simulink model "enginePistonPropC172p"  (R2026a)
settings: Solver=FixedStepAuto  FixedStep=0.004
settings Model: Creator=Edison Altamirano  LastModifiedBy=Edison Altamirano

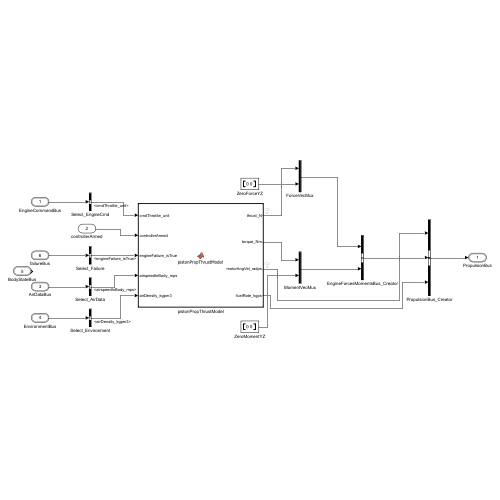
[thumbnail: Simulink's stored preview of the top-level diagram]
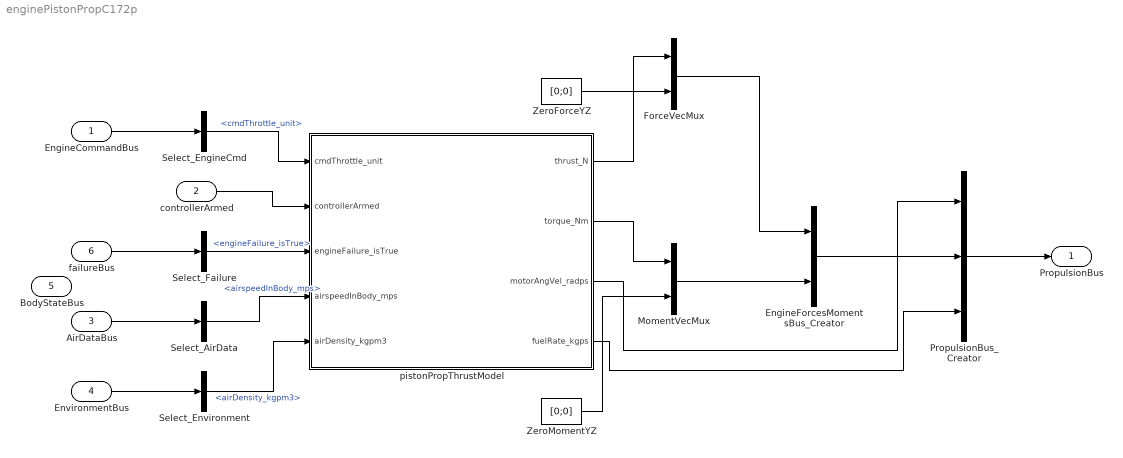
== system enginePistonPropC172p ==
  EngineCommandBus : Inport  OutDataTypeStr=Bus: EngineCommandBus
  controllerArmed : Inport  Port=2
  AirDataBus : Inport  Port=3  OutDataTypeStr=Bus: AirDataBus
  EnvironmentBus : Inport  Port=4  OutDataTypeStr=Bus: EnvironmentBus
  BodyStateBus : Inport  Port=5  OutDataTypeStr=Bus: BodyStateBus
  failureBus : Inport  Port=6  OutDataTypeStr=Bus: FailureBus
  EngineForcesMomentsBus_Creator : BusCreator  Inputs=2  OutDataTypeStr=Bus: ComponentForcesMomentsBus
  ForceVecMux : Mux  Inputs=2
  MomentVecMux : Mux  Inputs=2
  PropulsionBus_Creator : BusCreator  Inputs=3  OutDataTypeStr=Bus: PropulsionBus
  Select_AirData : BusSelector  OutputSignals=airspeedInBody_mps
  Select_EngineCmd : BusSelector  OutputSignals=cmdThrottle_unit
  Select_Environment : BusSelector  OutputSignals=AirEnvironment.airDensity_kgpm3
  Select_Failure : BusSelector  OutputSignals=engineFailure_isTrue
  ZeroForceYZ : Constant  Value=[0;0]
  ZeroMomentYZ : Constant  Value=[0;0]
  pistonPropThrustModel : MATLAB Function  TreatAsAtomicUnit=on
  PropulsionBus : Outport  OutDataTypeStr=Bus: PropulsionBus
  wires:
  EngineCommandBus/1 -> Select_EngineCmd/1
  Select_Failure/1 -> pistonPropThrustModel/3(engineFailure_isTrue)  "<engineFailure_isTrue>"
  AirDataBus/1 -> Select_AirData/1
  EnvironmentBus/1 -> Select_Environment/1
  pistonPropThrustModel/2(torque_Nm) -> MomentVecMux/1
  failureBus/1 -> Select_Failure/1
  Select_EngineCmd/1 -> pistonPropThrustModel/1(cmdThrottle_unit)  "<cmdThrottle_unit>"
  Select_AirData/1 -> pistonPropThrustModel/4(airspeedInBody_mps)  "<airspeedInBody_mps>"
  controllerArmed/1 -> pistonPropThrustModel/2(controllerArmed)
  PropulsionBus_Creator/1 -> PropulsionBus/1
  Select_Environment/1 -> pistonPropThrustModel/5(airDensity_kgpm3)  "<airDensity_kgpm3>"
  ZeroForceYZ/1 -> ForceVecMux/2
  pistonPropThrustModel/1(thrust_N) -> ForceVecMux/1
  pistonPropThrustModel/3(motorAngVel_radps) -> PropulsionBus_Creator/1
  pistonPropThrustModel/4(fuelRate_kgps) -> PropulsionBus_Creator/3
  ZeroMomentYZ/1 -> MomentVecMux/2
  ForceVecMux/1 -> EngineForcesMomentsBus_Creator/1
  MomentVecMux/1 -> EngineForcesMomentsBus_Creator/2
  EngineForcesMomentsBus_Creator/1 -> PropulsionBus_Creator/2

== matlab function enginePistonPropC172p/pistonPropThrustModel ==
  data: cmdThrottle_unit input; thrust_N output; controllerArmed input; engineFailure_isTrue input; airspeedInBody_mps input; airDensity_kgpm3 input; torque_Nm output; motorAngVel_radps output; fuelRate_kgps output
function [thrust_N, torque_Nm, motorAngVel_radps, fuelRate_kgps] = pistonPropThrustModel(cmdThrottle_unit, controllerArmed, engineFailure_isTrue, airspeedInBody_mps, airDensity_kgpm3)
%#codegen
persistent omega_radps_state;
if isempty(omega_radps_state)
    omega_radps_state = 0;
end

% Real Lycoming IO-320 limits (jsbsim/engine/eng_io320.xml) and Fixed-Pitch 75in prop tables
% (jsbsim/engine/prop_75in2f.xml) -- see vehicle/common/setUpActuators.m 'c172p' case for
% sourcing. Constants inlined (not read from vehicleParams) per the same MATLAB-Function-block
% constraint documented in optimAeroPX4SIL/CLAUDE.md section 3. KEEP IN SYNC BY HAND with
% setUpActuators.m if changed.
idleRPM = 550;
maxRPM = 2700;
maxPower_W = 160 * 745.7;
bsfc_lb_per_hp_hr = 0.32;
tauEngine_s = 1.0;
Ts_s = 0.01;
D_m = 75 * 0.0254;
J_bkpts_CT = [0.0 0.1 0.2 0.3 0.4 0.5 0.6 0.7 0.8 0.9 1.0 1.1 1.2 1.3 1.4 1.5 1.6 1.7 1.8 1.9 2.0 2.1 2.2 2.3 5.0];
CT_data    = [0.073 0.073 0.072 0.071 0.069 0.066 0.062 0.055 0.045 0.034 0.024 0.013 -0.006 -0.013 -0.024 -0.034 -0.045 -0.055 -0.062 -0.066 -0.069 -0.071 -0.072 -0.073 -0.073];
J_bkpts_CP = [0.0 0.1 0.2 0.3 0.4 0.5 0.6 0.7 0.8 0.9 1.0 1.1 1.2 1.3 1.4 1.5 1.6 1.7 1.8 1.9 2.0 2.1 2.2 2.3 2.4 5.0];
CP_data    = [0.0660 0.0700 0.0700 0.0660 0.0600 0.0530 0.0501 0.0469 0.0426 0.0360 0.0282 0.0191 0.0155 0.0191 0.0282 0.0360 0.0426 0.0469 0.0501 0.0516 0.0525 0.0525 0.0522 0.0511 0.0504 0.0493];

engineRunning = controllerArmed && ~engineFailure_isTrue;
if engineRunning
    throttleCmd_nd = max(min(cmdThrottle_unit, 1), 0);
    targetRPM = idleRPM + (maxRPM - idleRPM) * throttleCmd_nd;
else
    throttleCmd_nd = 0;
    targetRPM = 0;
end
targetOmega_radps = targetRPM * 2 * pi / 60;

alpha = Ts_s / (tauEngine_s + Ts_s);
omega_radps_state = omega_radps_state + alpha * (targetOmega_radps - omega_radps_state);
motorAngVel_radps = omega_radps_state;

n_rps = motorAngVel_radps / (2 * pi);
V_mps = norm(airspeedInBody_mps);
if n_rps > 1e-3
    J_nd = V_mps / (n_rps * D_m);
else
    J_nd = 0;
end
J_nd = max(min(J_nd, 3.0), 0);

Ct = interp1(J_bkpts_CT, CT_data, J_nd, 'linear', 'extrap');
Cp = interp1(J_bkpts_CP, CP_data, J_nd, 'linear', 'extrap');

thrust_N = Ct * airDensity_kgpm3 * n_rps^2 * D_m^4;
power_W = Cp * airDensity_kgpm3 * n_rps^3 * D_m^5;
power_W = min(power_W, maxPower_W);
if motorAngVel_radps > 1e-3
    torque_Nm = -power_W / motorAngVel_radps;
else
    torque_Nm = 0;
end

% bsfc-based fuel flow estimate (telemetry only -- see file header, this SIL never feeds
% fuelRate_kgps back into vehicle mass for ANY vehicle, not just this one).
power_hp = power_W / 745.7;
fuelRate_kgps = bsfc_lb_per_hp_hr * power_hp / 3600 * 0.453592;
end
